simulink model "TankSystem"  (R2020a)
settings: Solver=ode45  StartTime=0.0  StopTime=500  RelTol=1e-3  EnableMultiTasking=on
PreLoadFcn:
  | Initialize
StopFcn:
  | Plot_and_save
undefined symbols (not defined in the file or in its folder): AnalogToDigital, P, PlotTanks, PlotTanks1, PlotTanks2, SendEmbededData, SendEmbededData2, SendEmbededData3
libraries: simulink x9
settings Model: EnablePacing=on  Creator=tsladeche  LastModifiedBy=Asus_EliTe
settings DataIOCC: LimitDataPoints=on  SaveFormat=Array  ReturnWorkspaceOutputs=off
settings OptimizationCC: ExpressionDepthLimit=2147483647  LifeSpan=inf
settings DebuggingCC: UnderspecifiedInitializationDetection=Classic  MergeDetectMultiDrivingBlocksExec=none  SolverPrmCheckMsg=warning  FcnCallInpInsideContextMsg=warning  StateNameClashWarn=warning  SFUnexpectedBacktrackingDiag=warning  SFNoUnconditionalDefaultTransitionDiag=warning  SFExecutionAtInitializationDiag=none  ArithmeticOperatorsInVariantConditions=warning
settings HardwareCC: ProdBitPerPointer=32  ProdBitPerSizeT=32  ProdBitPerPtrDiffT=32  ProdLargestAtomicFloat=None  ProdIntDivRoundTo=Undefined  ProdEndianess=Unspecified  ProdWordSize=32  ProdHWDeviceType=32-bit Generic
settings ModelReferenceCC: PropagateSignalLabelsOutOfModel=off
settings SFSimCC: SimUseLocalCustomCode=off  CustomCodeUndefinedFunction=UseInterfaceOnly
settings RTWCC: RTWUseLocalCustomCode=off
settings CodeAppCC: StateflowObjectComments=on
settings GRTTargetCC: TargetLangStandard=C89/C90 (ANSI)  CombineOutputUpdateFcns=off  GRTInterface=on
settings ConfigComp: CovMetricSettings=dw  CovHtmlReporting=on  CovSaveCumulativeToWorkspaceVar=on  CovSaveSingleToWorkspaceVar=on  CovExternalEMLEnable=off  CovSFcnEnable=off

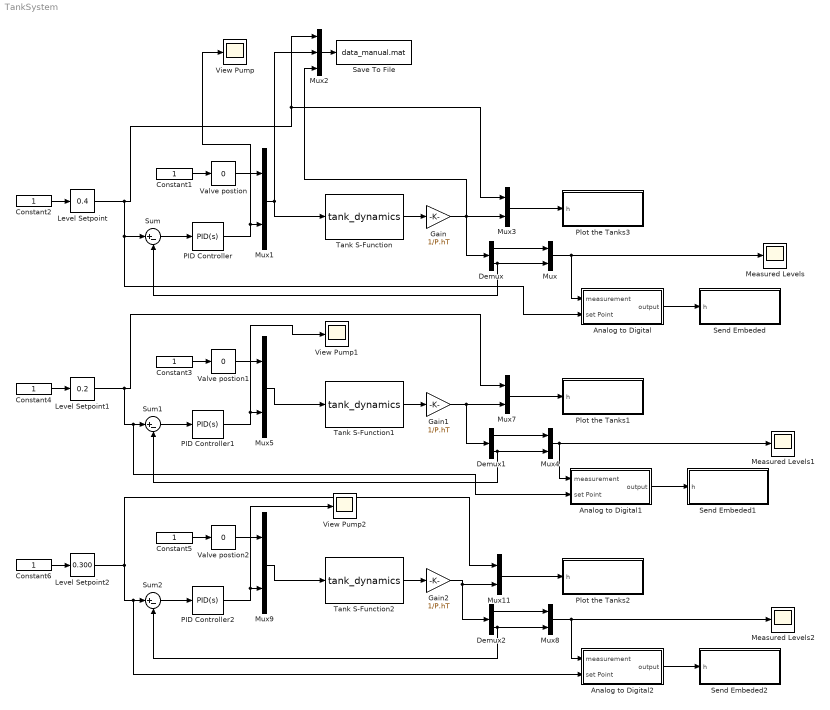
== system TankSystem ==
  Analog to Digital : Subsystem
  Analog to Digital1 : Subsystem
  Analog to Digital2 : Subsystem
  Constant1 : Constant  SampleTime=0.1
  Constant2 : Constant  SampleTime=0.1
  Constant{3..6} (4 alike) : Constant
  Demux : Demux  Outputs=2
  Demux1 : Demux  Outputs=2
  Demux2 : Demux  Outputs=2
  Gain : Gain  Gain=1/P.hT
  Gain1 : Gain  Gain=1/P.hT
  Gain2 : Gain  Gain=1/P.hT
  Level Setpoint : simulink/Math Operations/Slider Gain  gain=0.4  low=0  high=1
  Level Setpoint1 : simulink/Math Operations/Slider Gain  gain=0.2  low=0  high=1
  Level Setpoint2 : simulink/Math Operations/Slider Gain  gain=0.300  low=0  high=1
  Measured Levels : Scope
  Measured Levels1 : Scope
  Measured Levels2 : Scope
  Mux{,1,3..5,7..9,11} (9 alike) : Mux  Inputs=2
  Mux2 : Mux  Inputs=3
  PID Controller : simulink/Continuous/PID Controller  Controller=PID  Form=Parallel  TimeDomain=Continuous-time  UseExternalTs=off  SampleTime=-1  IntegratorMethod=Forward Euler  FilterMethod=Forward Euler  ControllerParametersSource=internal  P=5  I=5/(1.4*142)  D=3  UseFilter=on  N=100  TunerSelectOption=Transfer Function Based (PID Tuner App)  InitialConditionSource=internal  InitialConditionForIntegrator=0  InitialConditionForFilter=0  DifferentiatorICPrevScaledInput=0  ExternalReset=none  TrackingMode=off  Kt=1  LimitOutput=off  UpperSaturationLimit=inf  LowerSaturationLimit=-inf  LinearizeAsGain=on  AntiWindupMode=none  Kb=1  POutMin=[]  POutMax=[]  IOutMin=[]  IOutMax=[]  DOutMin=[]  DOutMax=[]  NOutMin=[]  NOutMax=[]  SumOutMin=[]  SumOutMax=[]  SaturationOutMin=[]  SaturationOutMax=[]  PParamMin=[]  PParamMax=[]  IParamMin=[]  IParamMax=[]  DParamMin=[]  DParamMax=[]  NParamMin=[]  NParamMax=[]  KbParamMin=[]  KbParamMax=[]  KtParamMin=[]  KtParamMax=[]  KbOutMin=[]  KbOutMax=[]  KtOutMin=[]  KtOutMax=[]  IntegratorOutMin=[]  IntegratorOutMax=[]  FilterOutMin=[]  FilterOutMax=[]  SumI1OutMin=[]  SumI1OutMax=[]  SumI2OutMin=[]  SumI2OutMax=[]  SumI3OutMin=[]  SumI3OutMax=[]  SumI4OutMin=[]  SumI4OutMax=[]  SumDOutMin=[]  SumDOutMax=[]  DifferentiatorOutMin=[]  DifferentiatorOutMax=[]  FilterDiffOutCoefMin=[]  FilterDiffOutCoefMax=[]  ReciprocalOutMin=[]  ReciprocalOutMax=[]  SumDenOutMin=[]  SumDenOutMax=[]  SumNumOutMin=[]  SumNumOutMax=[]  DivideOutMin=[]  DivideOutMax=[]  UdiffTsProdOutMin=[]  UdiffTsProdOutMax=[]  NTsProdOutMin=[]  NTsProdOutMax=[]  UintegralTsProdOutMin=[]  UintegralTsProdOutMax=[]  UngainTsProdOutMin=[]  UngainTsProdOutMax=[]  IntegratorContinuousStateAttributes=''  IntegratorStateMustResolveToSignalObject=off  IntegratorRTWStateStorageClass=Auto  FilterContinuousStateAttributes=''  FilterStateMustResolveToSignalObject=off  FilterRTWStateStorageClass=Auto  ParallelPVariant=InternalParameters  IdealPVariant=Disabled  IVariant=InternalParameters  DVariant=InternalParameters  IntegratorVariant=Continuous  SatVariant=Disabled  AWVariant=Passthrough  PCopyVariant=Disabled  TRVariant=Disabled  FdbkBlocksVariant=Forward  IdealPFdbkVariant=Disabled  SatFdbkVariant=Disabled  DerivativeFilterVariant=ContFilter  NVariant=InternalParameters  NCopyVariant=Disabled  FilterICVariant=InternalICsFilter  IntegratorICVariant=InternalICs  ExternalResetVariant=Disabled  TRSumVariant=Passthrough  SumFdbkVariant=Disabled  SumVariant=Sum_PID  TsampFilterVariant=InternalTs  TsampNgainVariant=Passthrough  TsampIntegralVariant=Passthrough
  PID Controller1 : simulink/Continuous/PID Controller  Controller=PID  Form=Parallel  TimeDomain=Continuous-time  UseExternalTs=off  SampleTime=-1  IntegratorMethod=Forward Euler  FilterMethod=Forward Euler  ControllerParametersSource=internal  P=5  I=5/(1.4*142)  D=3  UseFilter=on  N=100  TunerSelectOption=Transfer Function Based (PID Tuner App)  InitialConditionSource=internal  InitialConditionForIntegrator=0  InitialConditionForFilter=0  DifferentiatorICPrevScaledInput=0  ExternalReset=none  TrackingMode=off  Kt=1  LimitOutput=off  UpperSaturationLimit=inf  LowerSaturationLimit=-inf  LinearizeAsGain=on  AntiWindupMode=none  Kb=1  POutMin=[]  POutMax=[]  IOutMin=[]  IOutMax=[]  DOutMin=[]  DOutMax=[]  NOutMin=[]  NOutMax=[]  SumOutMin=[]  SumOutMax=[]  SaturationOutMin=[]  SaturationOutMax=[]  PParamMin=[]  PParamMax=[]  IParamMin=[]  IParamMax=[]  DParamMin=[]  DParamMax=[]  NParamMin=[]  NParamMax=[]  KbParamMin=[]  KbParamMax=[]  KtParamMin=[]  KtParamMax=[]  KbOutMin=[]  KbOutMax=[]  KtOutMin=[]  KtOutMax=[]  IntegratorOutMin=[]  IntegratorOutMax=[]  FilterOutMin=[]  FilterOutMax=[]  SumI1OutMin=[]  SumI1OutMax=[]  SumI2OutMin=[]  SumI2OutMax=[]  SumI3OutMin=[]  SumI3OutMax=[]  SumI4OutMin=[]  SumI4OutMax=[]  SumDOutMin=[]  SumDOutMax=[]  DifferentiatorOutMin=[]  DifferentiatorOutMax=[]  FilterDiffOutCoefMin=[]  FilterDiffOutCoefMax=[]  ReciprocalOutMin=[]  ReciprocalOutMax=[]  SumDenOutMin=[]  SumDenOutMax=[]  SumNumOutMin=[]  SumNumOutMax=[]  DivideOutMin=[]  DivideOutMax=[]  UdiffTsProdOutMin=[]  UdiffTsProdOutMax=[]  NTsProdOutMin=[]  NTsProdOutMax=[]  UintegralTsProdOutMin=[]  UintegralTsProdOutMax=[]  UngainTsProdOutMin=[]  UngainTsProdOutMax=[]  IntegratorContinuousStateAttributes=''  IntegratorStateMustResolveToSignalObject=off  IntegratorRTWStateStorageClass=Auto  FilterContinuousStateAttributes=''  FilterStateMustResolveToSignalObject=off  FilterRTWStateStorageClass=Auto  ParallelPVariant=InternalParameters  IdealPVariant=Disabled  IVariant=InternalParameters  DVariant=InternalParameters  IntegratorVariant=Continuous  SatVariant=Disabled  AWVariant=Passthrough  PCopyVariant=Disabled  TRVariant=Disabled  FdbkBlocksVariant=Forward  IdealPFdbkVariant=Disabled  SatFdbkVariant=Disabled  DerivativeFilterVariant=ContFilter  NVariant=InternalParameters  NCopyVariant=Disabled  FilterICVariant=InternalICsFilter  IntegratorICVariant=InternalICs  ExternalResetVariant=Disabled  TRSumVariant=Passthrough  SumFdbkVariant=Disabled  SumVariant=Sum_PID  TsampFilterVariant=InternalTs  TsampNgainVariant=Passthrough  TsampIntegralVariant=Passthrough
  PID Controller2 : simulink/Continuous/PID Controller  Controller=PID  Form=Parallel  TimeDomain=Continuous-time  UseExternalTs=off  SampleTime=-1  IntegratorMethod=Forward Euler  FilterMethod=Forward Euler  ControllerParametersSource=internal  P=5  I=5/(1.4*142)  D=3  UseFilter=on  N=100  TunerSelectOption=Transfer Function Based (PID Tuner App)  InitialConditionSource=internal  InitialConditionForIntegrator=0  InitialConditionForFilter=0  DifferentiatorICPrevScaledInput=0  ExternalReset=none  TrackingMode=off  Kt=1  LimitOutput=off  UpperSaturationLimit=inf  LowerSaturationLimit=-inf  LinearizeAsGain=on  AntiWindupMode=none  Kb=1  POutMin=[]  POutMax=[]  IOutMin=[]  IOutMax=[]  DOutMin=[]  DOutMax=[]  NOutMin=[]  NOutMax=[]  SumOutMin=[]  SumOutMax=[]  SaturationOutMin=[]  SaturationOutMax=[]  PParamMin=[]  PParamMax=[]  IParamMin=[]  IParamMax=[]  DParamMin=[]  DParamMax=[]  NParamMin=[]  NParamMax=[]  KbParamMin=[]  KbParamMax=[]  KtParamMin=[]  KtParamMax=[]  KbOutMin=[]  KbOutMax=[]  KtOutMin=[]  KtOutMax=[]  IntegratorOutMin=[]  IntegratorOutMax=[]  FilterOutMin=[]  FilterOutMax=[]  SumI1OutMin=[]  SumI1OutMax=[]  SumI2OutMin=[]  SumI2OutMax=[]  SumI3OutMin=[]  SumI3OutMax=[]  SumI4OutMin=[]  SumI4OutMax=[]  SumDOutMin=[]  SumDOutMax=[]  DifferentiatorOutMin=[]  DifferentiatorOutMax=[]  FilterDiffOutCoefMin=[]  FilterDiffOutCoefMax=[]  ReciprocalOutMin=[]  ReciprocalOutMax=[]  SumDenOutMin=[]  SumDenOutMax=[]  SumNumOutMin=[]  SumNumOutMax=[]  DivideOutMin=[]  DivideOutMax=[]  UdiffTsProdOutMin=[]  UdiffTsProdOutMax=[]  NTsProdOutMin=[]  NTsProdOutMax=[]  UintegralTsProdOutMin=[]  UintegralTsProdOutMax=[]  UngainTsProdOutMin=[]  UngainTsProdOutMax=[]  IntegratorContinuousStateAttributes=''  IntegratorStateMustResolveToSignalObject=off  IntegratorRTWStateStorageClass=Auto  FilterContinuousStateAttributes=''  FilterStateMustResolveToSignalObject=off  FilterRTWStateStorageClass=Auto  ParallelPVariant=InternalParameters  IdealPVariant=Disabled  IVariant=InternalParameters  DVariant=InternalParameters  IntegratorVariant=Continuous  SatVariant=Disabled  AWVariant=Passthrough  PCopyVariant=Disabled  TRVariant=Disabled  FdbkBlocksVariant=Forward  IdealPFdbkVariant=Disabled  SatFdbkVariant=Disabled  DerivativeFilterVariant=ContFilter  NVariant=InternalParameters  NCopyVariant=Disabled  FilterICVariant=InternalICsFilter  IntegratorICVariant=InternalICs  ExternalResetVariant=Disabled  TRSumVariant=Passthrough  SumFdbkVariant=Disabled  SumVariant=Sum_PID  TsampFilterVariant=InternalTs  TsampNgainVariant=Passthrough  TsampIntegralVariant=Passthrough
  Plot the Tanks1 : Subsystem
  Plot the Tanks2 : Subsystem
  Plot the Tanks3 : Subsystem
  Save To File : ToFile  Filename=data_manual.mat  MatrixName=tanks  SampleTime=1
  Send Embeded : Subsystem
  Send Embeded1 : Subsystem
  Send Embeded2 : Subsystem
  Sum : Sum  Inputs=|+-
  Sum1 : Sum  Inputs=|+-
  Sum2 : Sum  Inputs=|+-
  Tank S-Function : S-Function  FunctionName=tank_dynamics  Parameters=P  SFunctionDeploymentMode=off  EnableBusSupport=off
  Tank S-Function1 : S-Function  FunctionName=tank_dynamics  Parameters=P1  SFunctionDeploymentMode=off  EnableBusSupport=off
  Tank S-Function2 : S-Function  FunctionName=tank_dynamics  Parameters=P2  SFunctionDeploymentMode=off  EnableBusSupport=off
  Valve postion : simulink/Math Operations/Slider Gain  gain=0  low=0  high=1
  Valve postion1 : simulink/Math Operations/Slider Gain  gain=0  low=0  high=1
  Valve postion2 : simulink/Math Operations/Slider Gain  gain=0  low=0  high=1
  View Pump : Scope
  View Pump1 : Scope
  View Pump2 : Scope
  wires:
  Gain/1 -> Mux3/2, Demux/1, Mux2/3
  Tank S-Function/1 -> Gain/1
  Mux2/1 -> Save To File/1
  Constant1/1 -> Valve postion/1
  Mux1/1 -> Mux2/2, Tank S-Function/1
  PID Controller/1 -> Mux1/2, View Pump/1
  Valve postion/1 -> Mux1/1
  Constant2/1 -> Level Setpoint/1
  Level Setpoint/1 -> Sum/1, Analog to Digital/2(set Point), Mux3/1, Mux2/1
  Mux/1 -> Analog to Digital/1(measurement), Measured Levels/1
  Demux/1 -> Mux/1
  Demux/2 -> Sum/2, Mux/2
  Sum/1 -> PID Controller/1
  Sum1/1 -> PID Controller1/1
  Demux1/2 -> Sum1/2, Mux4/2
  Constant4/1 -> Level Setpoint1/1
  Demux1/1 -> Mux4/1
  Gain1/1 -> Mux7/2, Demux1/1
  Constant3/1 -> Valve postion1/1
  Mux4/1 -> Analog to Digital1/1(measurement), Measured Levels1/1
  Tank S-Function1/1 -> Gain1/1
  PID Controller1/1 -> Mux5/2, View Pump1/1
  Level Setpoint1/1 -> Analog to Digital1/2(set Point), Sum1/1, Mux7/1
  Valve postion1/1 -> Mux5/1
  Mux5/1 -> Tank S-Function1/1
  Sum2/1 -> PID Controller2/1
  Demux2/2 -> Sum2/2, Mux8/2
  Constant6/1 -> Level Setpoint2/1
  Demux2/1 -> Mux8/1
  Gain2/1 -> Mux11/2, Demux2/1
  Constant5/1 -> Valve postion2/1
  Mux8/1 -> Analog to Digital2/1(measurement), Measured Levels2/1
  Tank S-Function2/1 -> Gain2/1
  PID Controller2/1 -> Mux9/2, View Pump2/1
  Level Setpoint2/1 -> Analog to Digital2/2(set Point), Sum2/1, Mux11/1
  Valve postion2/1 -> Mux9/1
  Mux9/1 -> Tank S-Function2/1
  Mux11/1 -> Plot the Tanks2/1(h)
  Mux7/1 -> Plot the Tanks1/1(h)
  Mux3/1 -> Plot the Tanks3/1(h)
  Analog to Digital/1(output) -> Send Embeded/1(h)
  Analog to Digital1/1(output) -> Send Embeded1/1(h)
  Analog to Digital2/1(output) -> Send Embeded2/1(h)

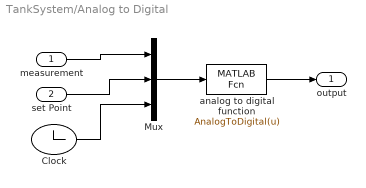
== system TankSystem/Analog to Digital ==
  measurement : Inport
  set Point : Inport  Port=2
  Clock : Clock
  Mux : Mux  Inputs=3
  analog to digital function : MATLABFcn  MATLABFcn=AnalogToDigital(u)  OutputDimensions=1  SampleTime=.05
  output : Outport
  wires:
  Mux/1 -> analog to digital function/1
  Clock/1 -> Mux/3
  measurement/1 -> Mux/1
  analog to digital function/1 -> output/1
  set Point/1 -> Mux/2

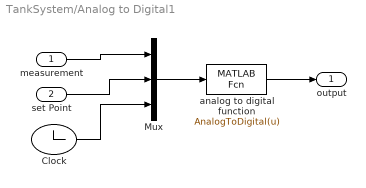
== system TankSystem/Analog to Digital1 ==
  measurement : Inport
  set Point : Inport  Port=2
  Clock : Clock
  Mux : Mux  Inputs=3
  analog to digital function : MATLABFcn  MATLABFcn=AnalogToDigital(u)  OutputDimensions=1  SampleTime=.05
  output : Outport
  wires:
  Mux/1 -> analog to digital function/1
  Clock/1 -> Mux/3
  measurement/1 -> Mux/1
  analog to digital function/1 -> output/1
  set Point/1 -> Mux/2

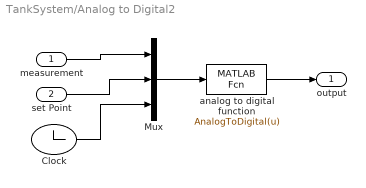
== system TankSystem/Analog to Digital2 ==
  measurement : Inport
  set Point : Inport  Port=2
  Clock : Clock
  Mux : Mux  Inputs=3
  analog to digital function : MATLABFcn  MATLABFcn=AnalogToDigital(u)  OutputDimensions=1  SampleTime=.05
  output : Outport
  wires:
  Mux/1 -> analog to digital function/1
  Clock/1 -> Mux/3
  measurement/1 -> Mux/1
  analog to digital function/1 -> output/1
  set Point/1 -> Mux/2

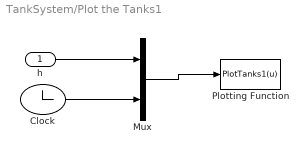
== system TankSystem/Plot the Tanks1 ==
  h : Inport
  Clock : Clock
  Mux : Mux  Inputs=2
  Plotting Function : MATLABFcn  MATLABFcn=PlotTanks1(u)  OutputDimensions=0  SampleTime=.05
  wires:
  Mux/1 -> Plotting Function/1
  Clock/1 -> Mux/2
  h/1 -> Mux/1

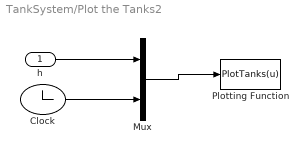
== system TankSystem/Plot the Tanks2 ==
  h : Inport
  Clock : Clock
  Mux : Mux  Inputs=2
  Plotting Function : MATLABFcn  MATLABFcn=PlotTanks(u)  OutputDimensions=0  SampleTime=.05
  wires:
  Mux/1 -> Plotting Function/1
  Clock/1 -> Mux/2
  h/1 -> Mux/1

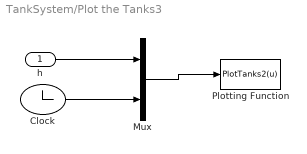
== system TankSystem/Plot the Tanks3 ==
  h : Inport
  Clock : Clock
  Mux : Mux  Inputs=2
  Plotting Function : MATLABFcn  MATLABFcn=PlotTanks2(u)  OutputDimensions=0  SampleTime=.05
  wires:
  Mux/1 -> Plotting Function/1
  Clock/1 -> Mux/2
  h/1 -> Mux/1

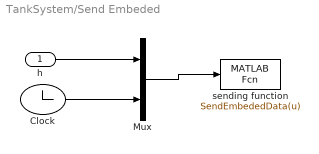
== system TankSystem/Send Embeded ==
  h : Inport
  Clock : Clock
  Mux : Mux  Inputs=2
  sending function : MATLABFcn  MATLABFcn=SendEmbededData(u)  OutputDimensions=0  SampleTime=.05
  wires:
  Mux/1 -> sending function/1
  Clock/1 -> Mux/2
  h/1 -> Mux/1

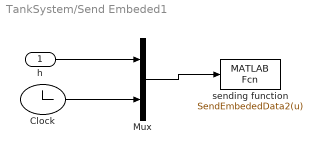
== system TankSystem/Send Embeded1 ==
  h : Inport
  Clock : Clock
  Mux : Mux  Inputs=2
  sending function : MATLABFcn  MATLABFcn=SendEmbededData2(u)  OutputDimensions=0  SampleTime=.05
  wires:
  Mux/1 -> sending function/1
  Clock/1 -> Mux/2
  h/1 -> Mux/1

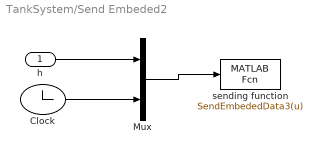
== system TankSystem/Send Embeded2 ==
  h : Inport
  Clock : Clock
  Mux : Mux  Inputs=2
  sending function : MATLABFcn  MATLABFcn=SendEmbededData3(u)  OutputDimensions=0  SampleTime=.05
  wires:
  Mux/1 -> sending function/1
  Clock/1 -> Mux/2
  h/1 -> Mux/1
